simulink model "DCC_DTC_v0"  (R2023b)
settings: Solver=VariableStepDiscrete  StartTime=0.0  StopTime=10.0  RelTol=1e-3
libraries: spsDCVoltageSourceLib x1, spsGroundLib x1, spsPermanentMagnetSynchronousMachineLib x1, spsThreePhaseVIMeasurementLib x1, spsUniversalBridgeLib x1, spspowerguiLib x1
settings Model: Creator=rainy  LastModifiedBy=rainy

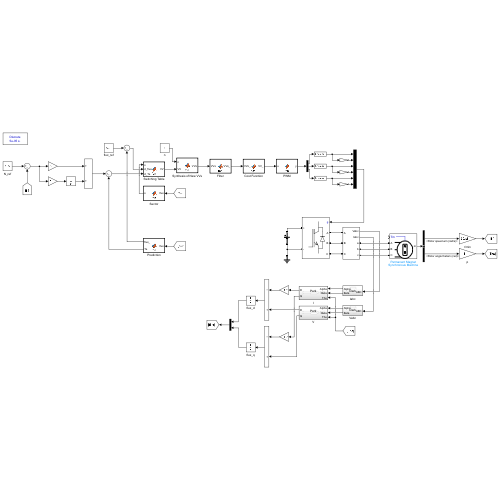
[thumbnail: Simulink's stored preview of the top-level diagram]
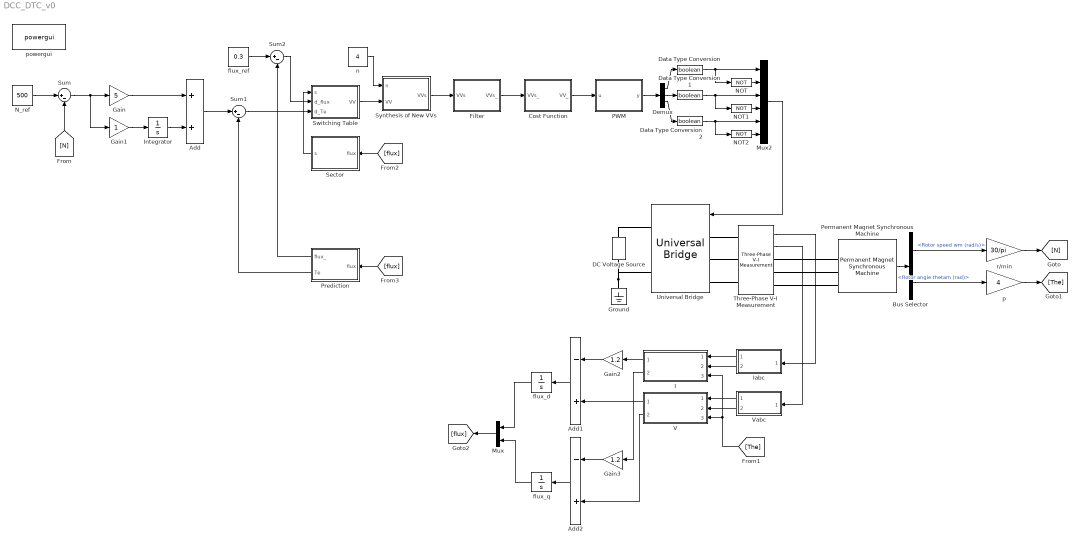
== system DCC_DTC_v0 ==
  Add : Sum
  Add1 : Sum  Inputs=-+
  Add2 : Sum  Inputs=-+
  Bus Selector : BusSelector  OutputSignals=Rotor speed wm (rad/s),Rotor angle thetam (rad)
  Cost Function : MATLAB Function  TreatAsAtomicUnit=on
  DC Voltage Source : spsDCVoltageSourceLib/DC Voltage Source  Amplitude=311  Measurements=Voltage
  Data Type Conversion : DataTypeConversion  OutDataTypeStr=boolean  SaturateOnIntegerOverflow=off  RndMeth=Floor
  Data Type Conversion1 : DataTypeConversion  OutDataTypeStr=boolean  SaturateOnIntegerOverflow=off  RndMeth=Floor
  Data Type Conversion2 : DataTypeConversion  OutDataTypeStr=boolean  SaturateOnIntegerOverflow=off  RndMeth=Floor
  Demux : Demux  Outputs=3
  Filter : MATLAB Function  TreatAsAtomicUnit=on
  Gain : Gain  Gain=5
  Gain1 : Gain
  Gain2 : Gain  Gain=1.2
  Gain3 : Gain  Gain=1.2
  Ground : spsGroundLib/Ground  LConnTagsString=a
  I : Subsystem  ReferencedSubsystem=Park
  Iabc : Subsystem  ReferencedSubsystem=Clark
  Integrator : Integrator
  Mux : Mux  Inputs=2
  Mux2 : Mux  Inputs=6
  NOT : Logic  Operator=NOT  IconShape=distinctive  AllPortsSameDT=off  OutDataTypeStr=boolean
  NOT1 : Logic  Operator=NOT  IconShape=distinctive  AllPortsSameDT=off  OutDataTypeStr=boolean
  NOT2 : Logic  Operator=NOT  IconShape=distinctive  AllPortsSameDT=off  OutDataTypeStr=boolean
  N_ref : Constant  Value=500
  PWM : MATLAB Function  TreatAsAtomicUnit=on
  Permanent Magnet Synchronous Machine : spsPermanentMagnetSynchronousMachineLib/Permanent Magnet Synchronous Machine  NbPhases=3  FluxDistribution=Sinusoidal  RotorType=Round  MechanicalLoad=Torque Tm  PresetModel=No  ShowDetailedParameters=on  MeasurementBus=off  Resistance=1.2  Inductance=8.5e-3  dqInductances=[8.5e-3,8.5e-3]  La=8.5e-3  MachineConstant=Flux linkage established by magnets (V.s)  Flux=0.175  VoltageCst=126.966  TorqueCst=1.05  Flat=120  Mechanical=[0.0008 0.0004924 4 0]  PolePairs=4  InitialConditions=[0,0, 0,0]  InitialConditions5ph=[0 0 0 0 0 0]  RefAngle=Aligned with phase A axis (original Park)  IterativeDiscreteModel=Trapezoidal non iterative  TsBlock=-1  TsPowergui=0
  Prediction : MATLAB Function  TreatAsAtomicUnit=on
  Sector : MATLAB Function  TreatAsAtomicUnit=on
  Sum : Sum  Inputs=|+-
  Sum1 : Sum  Inputs=|+-
  Sum2 : Sum  Inputs=|+-
  Switching Table : MATLAB Function  TreatAsAtomicUnit=on
  Synthesis of New VVs : MATLAB Function  TreatAsAtomicUnit=on
  Three-Phase V-I Measurement : spsThreePhaseVIMeasurementLib/Three-Phase V-I Measurement  VoltageMeasurement=phase-to-ground  SetLabelV=off  LabelV=Vabc  Vpu=off  VpuLL=off  CurrentMeasurement=yes  SetLabelI=off  LabelI=Iabc  Ipu=off  Pbase=100e6  Vbase=500e3  OutputType=Complex  PhasorSimulation=off  PSBequivalent=0
  Universal Bridge : spsUniversalBridgeLib/Universal Bridge  Arms=3  SnubberResistance=1e5  SnubberCapacitance=inf  Device=IGBT / Diodes  Ron=1e-3  Lon=0  ForwardVoltages="[  0  0  ]"  ForwardVoltage=0  GTOparameters=[ 10e-6 , 20e-6 ]  IGBTparameters=[ 1e-6 , 2e-6 ]  Measurements=None  Measurements_2=None  converterType=Rectifier
  V : Subsystem  ReferencedSubsystem=Park
  Vabc : Subsystem  ReferencedSubsystem=Clark
  flux_d : Integrator
  flux_q : Integrator
  flux_ref : Constant  Value=0.3
  n : Constant  Value=4
  p : Gain  Gain=4
  powergui : spspowerguiLib/powergui  Priority=1  SimulationMode=Discrete  SampleTime=50e-6  frequency=60  Iterations=50  frequencyindice=0  Pbase=100e6  ErrMax=1e-4  UnitsV=kV  UnitsW=MW  buscounter=0  FunctionMessages=off  echomessages=off  EnableUseOfTLC=off  CurrentSourceSwitches=off  DisableSnubberDevices=off  DisableRonSwitches=off  DisableVfSwitches=off  DisplayEquations=off  AutomaticDiscreteSolvers=off  SolverType=Tustin/Backward Euler (TBE)  Interpol=off  ExternalGateDelay=off  methode=off  Ts=100  x0status=blocks  SPID=on  SwTol=0  HookPort=off  NonlinearTolerance=1e-4  nMaxIteration=100  ContinueOnMaxIteration=off  RestoreLinks=warning  ResistiveCurrentMeasurement=off  Frange=[0:2:500]  Ylog=off  Xlog=on  ShowGrid=off  save=off  variable=ZData  structure=0  ZoomFFT=off  StartTime=0.0  cycles=1  DisplayStyle=1  fundamental=60  FreqAxis=off  MaxFrequency=1000  frequencyindicesteady=1  RmsSteady=1  display=off
  r/min : Gain  Gain=30/pi
  wires:
  N_ref/1 -> Sum/1
  Sum/1 -> Gain/1, Gain1/1
  Gain1/1 -> Integrator/1
  Gain/1 -> Add/1
  Integrator/1 -> Add/2
  Add/1 -> Sum1/1
  flux_ref/1 -> Sum2/1
  Sum1/1 -> Switching Table/3(d_Te)
  Sum2/1 -> Switching Table/2(d_flux)
  Permanent Magnet Synchronous Machine/1 -> Bus Selector/1
  Bus Selector/1 -> r/min/1  "<Rotor speed wm (rad/s)>"
  V/1 -> Add1/2
  I/1 -> Gain2/1
  Vabc/2 -> V/2
  Three-Phase V-I Measurement/1 -> Iabc/1
  Vabc/1 -> V/1
  Three-Phase V-I Measurement/2 -> Vabc/1
  Gain2/1 -> Add1/1
  Add1/1 -> flux_d/1
  Iabc/1 -> I/1
  Iabc/2 -> I/2
  r/min/1 -> [N]
  [N] -> Sum/2
  Bus Selector/2 -> p/1  "<Rotor angle thetam (rad)>"
  [The] -> V/3, I/3
  Add2/1 -> flux_q/1
  Gain3/1 -> Add2/1
  V/2 -> Add2/2
  I/2 -> Gain3/1
  p/1 -> [The]
  Sector/1(s) -> Switching Table/1(s)
  Switching Table/1(VV) -> Synthesis of New VVs/2(VV)
  n/1 -> Synthesis of New VVs/1(n)
  Synthesis of New VVs/1(VVs) -> Filter/1(VVs)
  Filter/1(VVs_) -> Cost Function/1(VVs_)
  NOT1/1 -> Mux2/4
  Data Type Conversion2/1 -> NOT2/1, Mux2/5
  Mux2/1 -> Universal Bridge/1
  NOT2/1 -> Mux2/6
  Data Type Conversion/1 -> NOT/1, Mux2/1
  NOT/1 -> Mux2/2
  Data Type Conversion1/1 -> NOT1/1, Mux2/3
  Cost Function/1(VV_) -> PWM/1(u)
  Demux/1 -> Data Type Conversion/1
  Demux/2 -> Data Type Conversion1/1
  Demux/3 -> Data Type Conversion2/1
  PWM/1(y) -> Demux/1
  flux_d/1 -> Mux/1
  flux_q/1 -> Mux/2
  Mux/1 -> [flux]
  [flux] -> Sector/1(flux)
  [flux] -> Prediction/1(flux)
  Prediction/2(Te) -> Sum1/2
  Prediction/1(flux_) -> Sum2/2
  connections:
  Ground/LConn1 -- Universal Bridge/RConn2 -- DC Voltage Source/LConn1
  Permanent Magnet Synchronous Machine/LConn2 -- Three-Phase V-I Measurement/RConn2
  Permanent Magnet Synchronous Machine/LConn1 -- Three-Phase V-I Measurement/RConn1
  Universal Bridge/LConn3 -- Three-Phase V-I Measurement/LConn3
  Universal Bridge/LConn1 -- Three-Phase V-I Measurement/LConn1
  Universal Bridge/LConn2 -- Three-Phase V-I Measurement/LConn2
  DC Voltage Source/RConn1 -- Universal Bridge/RConn1
  Permanent Magnet Synchronous Machine/LConn3 -- Three-Phase V-I Measurement/RConn3

== matlab function DCC_DTC_v0/Sector ==
  data: flux input; s output
function s = fcn(flux)

% 将\psi_{\aplha}和\psi_{\beta}分解为三相
a1 = flux(1);
b1 = flux(1)*(-0.5) + sqrt(3)/2*flux(2);
c1 = flux(1)*(-0.5) - sqrt(3)/2*flux(2);

% a1 > 0，有扇区126
% b1 > 0，有扇区234
% c1 > 0，有扇区456
% n为a1 b1 c1中>0的个数，0 < n < 3
% 
% a b c | s
%-------|---
% 1 1 0 | 2
% 1 0 1 | 6
% 1 0 0 | 1
% 0 1 1 | 4
% 0 1 0 | 3
% 0 0 1 | 5

if(a1 > 0)
    a = 1;
else
    a = 0;
end

if(b1 > 0)
    b = 1;
else
    b = 0;
end

if(c1 > 0)
    c = 1;
else
    c = 0;
end

N = 4*a+2*b+c;

Sector_table=[5 3 4 1 6 2];

s = Sector_table(N);

== matlab function DCC_DTC_v0/Switching Table ==
  data: s input; d_flux input; d_Te input; VV output
function VV = fcn(s, d_flux, d_Te)

VV = u;

== matlab function DCC_DTC_v0/Prediction ==
  data: flux_ output; Te output; flux input
function [flux_, Te]= fcn(flux)

[flux_, Te] = u;

== matlab function DCC_DTC_v0/Synthesis of New VVs ==
  data: n input; VV input; VVs output
function VVs = fcn(n, VV)

VVs = u;

== matlab function DCC_DTC_v0/Filter ==
  data: VVs input; VVs_ output
function VVs_ = fcn(VVs)

VVs_ = u;

== matlab function DCC_DTC_v0/Cost Function ==
  data: VVs_ input; VV_ output
function VV_ = fcn(VVs_)

y = u;

== matlab function DCC_DTC_v0/PWM ==
  data: u input; y output
function y = fcn(u)

y = u;
